simulink model "simulink_exo1"  (R2014a)
settings: Solver=ode45  StartTime=0.0  StopTime=tf  RelTol=1e-3
values from neighbouring files (symbols this model uses):
  A = [0 1 ; 1 -2]    [TP1_exo1.m]
  B = [0 ; 1]    [TP1_exo1.m]
  Pin = flipud(Pout)    [TP1_exo1.m]
  Tin = flipud(Tout)    [TP1_exo1.m]
settings Model: Creator=m2rodeco_01  LastModifiedBy=Eugene Shulga
settings OptimizationCC: ExpressionDepthLimit=2147483647
settings DebuggingCC: UnderspecifiedInitializationDetection=Classic  StateNameClashWarn=warning

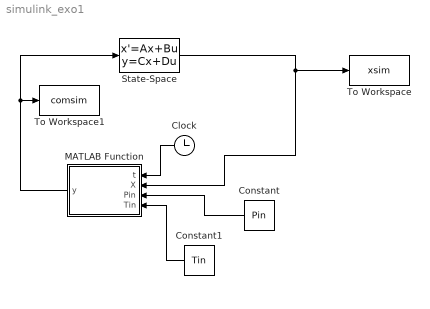
== system simulink_exo1 ==
  Clock : Clock
  Constant : Constant  Value=Pin
  Constant1 : Constant  Value=Tin
  MATLAB Function : MATLAB Function  TreatAsAtomicUnit=on
  State-Space : StateSpace  A=A  B=B  C=[1 0; 0 1]  D=[0;0]  X0=[2;1]
  To Workspace : ToWorkspace  VariableName=xsim  SaveFormat=Timeseries  SampleTime=-1
  To Workspace1 : ToWorkspace  VariableName=comsim  SaveFormat=Timeseries  SampleTime=-1
  wires:
  MATLAB Function/1(y) -> To Workspace1/1, State-Space/1
  Clock/1 -> MATLAB Function/1(t)
  Constant/1 -> MATLAB Function/3(Pin)
  Constant1/1 -> MATLAB Function/4(Tin)
  State-Space/1 -> To Workspace/1, MATLAB Function/2(X)

== matlab function simulink_exo1/MATLAB Function ==
  data: y output; t input; X input; Pin input; Tin input
function y = fcn(t,X,Pin,Tin)
%#codegen
    R=2;
    B=[0 ; 1];
    
    Pt=interp1(Tin,Pin,t);
    P=[Pt(1) Pt(2) ;Pt(3) Pt(4)];
    u=-R^(-1)*B'*P*X;
    y = u;
end
